simulink model "TestInSimulink"  (R2024b)
settings: Solver=FixedStepAuto  StartTime=0.0  StopTime=60.0  FixedStep=0.01  RelTol=1e-3
values from neighbouring files (symbols this model uses):
  DrivetrainEff = 0.95756    [TestInSimulink_prmts.m]
  Mode = 3    [TestInSimulink_prmts.m]
  Omega0 = 7.55    [TestInSimulink_prmts.m]
  rpm2radps = pi/30    (= 0.10471975512)    [TestInSimulink_prmts.m]
  SwingEq = 1/1836784*30/pi*1000    (= 0.00519892191216)    [TestInSimulink_prmts.m]
libraries: simulink x1
settings Model: Creator=valentinc  LastModifiedBy=valentinc
settings DebuggingCC: DebugExecutionForFMUViaOutOfProcess=on
settings RTWCC: GPUComputeCapability=3.5

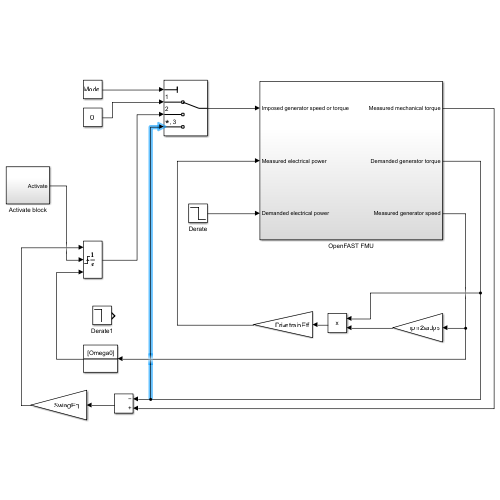
[thumbnail: Simulink's stored preview of the top-level diagram]
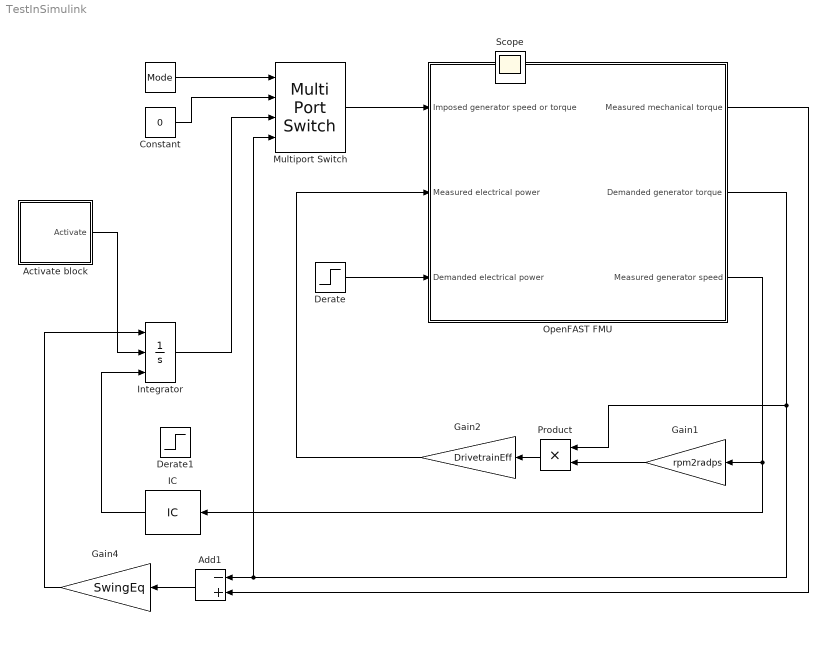
== system TestInSimulink ==
  " " : Constant  Value=Mode
  Activate block : Subsystem
  Add1 : Sum  Inputs=-+
  Constant : Constant  Value=0
  Derate : Step  Time=5  Before=2e4  After=1e4  SampleTime=0
  Derate1 : Step  Time=5  Before=19000  After=12000  SampleTime=0
  Gain1 : Gain  Gain=rpm2radps
  Gain2 : Gain  Gain=DrivetrainEff
  Gain4 : Gain  Gain=SwingEq
  IC : InitialCondition  Value=Omega0
  Integrator : Integrator  ExternalReset=rising  InitialConditionSource=external  InitialCondition=7.55
  Multiport Switch : MultiPortSwitch  SaturateOnIntegerOverflow=off  InputSameDT=off
  OpenFAST FMU : Subsystem
  Product : Product
  Scope : Scope
  wires:
  Product/1 -> Gain2/1
  Derate/1 -> OpenFAST FMU/3(Demanded electrical power)
  IC/1 -> Integrator/3
  Gain2/1 -> OpenFAST FMU/2(Measured electrical power)
  Gain1/1 -> Product/2
  OpenFAST FMU/3(Measured generator speed) -> Gain1/1, IC/1
  OpenFAST FMU/2(Demanded generator torque) -> Multiport Switch/4, Add1/1, Product/1
  Add1/1 -> Gain4/1
  Gain4/1 -> Integrator/1
  Activate block/1(Activate) -> Integrator/2
  " "/1 -> Multiport Switch/1
  Multiport Switch/1 -> OpenFAST FMU/1(Imposed generator speed or torque)
  Integrator/1 -> Multiport Switch/3
  OpenFAST FMU/1(Measured mechanical torque) -> Add1/2
  Constant/1 -> Multiport Switch/2

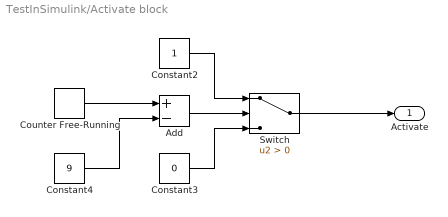
== system TestInSimulink/Activate block ==
  Add : Sum  Inputs=+-
  Constant2 : Constant
  Constant3 : Constant  Value=0
  Constant4 : Constant  Value=9
  Counter Free-Running : simulink/Sources/Counter Free-Running  NumBits=16  tsamp=-1
  Switch : Switch  Criteria=u2 > Threshold  SaturateOnIntegerOverflow=off  InputSameDT=off
  Activate : Outport
  wires:
  Constant2/1 -> Switch/1
  Constant4/1 -> Add/2
  Counter Free-Running/1 -> Add/1
  Add/1 -> Switch/2
  Constant3/1 -> Switch/3
  Switch/1 -> Activate/1

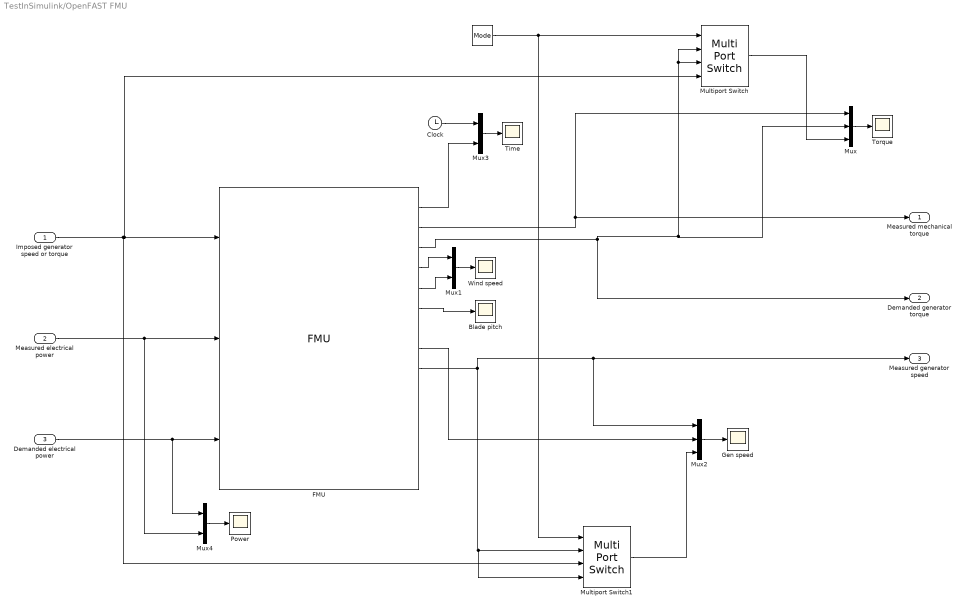
== system TestInSimulink/OpenFAST FMU ==
  Imposed generator speed or torque : Inport
  Measured electrical power : Inport  Port=2
  Demanded electrical power : Inport  Port=3
  "  " : Constant  Value=Mode
  Blade pitch : Scope
  Clock : Clock
  FMU : FMU  FMUName=fast.fmu  FMUDebugLogging=on  FMUMode=CoSimulation  FMUIsToleranceUsed=on  FMUSampleTime=0.01  FMUInitializeEnumObject=off  FMUCachedDialogLayout="{\"Geometry\":[2070,342,1033,905],\"ParameterColumnsWidthConfig\":\"{\\\"columns\\\":[{\\\"name\\\":\\\"Parameter\\\",\\\"width\\\":95},{\\\"name\\\":\\\"Value\\\",\\\"width\\\":59},{\\\"name\\\":\\\"Unit\\\",\\\"width\\\":49},{\\\"name\\\":\\\"Description\\\",\\\"width\\\":103}]}\",\"InputColumnsWidthConfig\":\"{\\\"columns\\\":[{\\\"name\\\":\\\"Name\\\",\\\"width\\\":63},{\\\"name\\\":\\\"Visibility\\\",\\\"width\\\":79},{\\\"name\\\":\\\"Start\\\",\\\"width\\\":52},{\\\"name\\\":\\\"Unit\\\",\\\"width\\\":49},{\\\"name\\\":\\\"Type Object\\\",\\\"width\\\":107}]}\",\"OutputColumnsWidthConfig\":\"{\\\"columns\\\":[{\\\"name\\\":\\\"Name\\\",\\\"width\\\":292},{\\\"name\\\":\\\"Visibility\\\",\\\"width\\\":79},{\\\"name\\\":\\\"Start\\\",\\\"width\\\":281},{\\\"name\\\":\\\"Unit\\\",\\\"width\\\":278},{\\\"name\\\":\\\"Type Object\\\",\\\"width\\\":337}]}\"}"  testNr=1002  timeStart=0  Mode=Mode  DebugPrmt=1  mask(FAST FMU [Co-Simulation, v2.0]){}
      mask Display:
      | disp('FAST FMU');
      | port_label('output',1,'Time');
      | port_label('output',2,'HSShftTq');
      | port_label('output',3,'GenTq');
      | port_label('output',4,'Wind1VelX');
      | port_label('output',5,'RtVAvgxh');
      | port_label('output',6,'BldPitch1');
      | port_label('output',7,'NacYaw');
      | port_label('output',8,'RefGenSpd');
      | port_label('output',9,'GenSpeed');
      | port_label('output',10,'RotSpeed');
      | port_label('output',11,'LSSGagPxa');
      | port_label('output',12,'Azimuth');
      | port_label('output',13,'GenAccel');
      | port_label('output',14,'YawBrTAxp');
      | port_label('input',1,'GenSpdOrTrq');
      | port_label('input',2,'GenPwr');
      | port_label('input',3,'ElecPwrCom');
  Gen speed : Scope
  Multiport Switch : MultiPortSwitch  SaturateOnIntegerOverflow=off  InputSameDT=off
  Multiport Switch1 : MultiPortSwitch  SaturateOnIntegerOverflow=off  InputSameDT=off
  Mux : Mux  Inputs=3
  Mux1 : Mux  Inputs=2
  Mux2 : Mux  Inputs=3
  Mux3 : Mux  Inputs=2
  Mux4 : Mux  Inputs=2
  Power : Scope
  Time : Scope
  Torque : Scope
  Wind speed : Scope
  Measured mechanical torque : Outport
  Demanded generator torque : Outport  Port=2
  Measured generator speed : Outport  Port=3
  wires:
  FMU/9 -> Mux2/1, Measured generator speed/1, Multiport Switch1/4, Multiport Switch1/2
  Demanded electrical power/1 -> Mux4/1, FMU/3
  Measured electrical power/1 -> Mux4/2, FMU/2
  FMU/3 -> Mux/2, Multiport Switch/3, Multiport Switch/2, Demanded generator torque/1
  FMU/2 -> Mux/1, Measured mechanical torque/1
  Mux/1 -> Torque/1
  FMU/6 -> Blade pitch/1
  FMU/4 -> Mux1/1
  FMU/5 -> Mux1/2
  Mux1/1 -> Wind speed/1
  FMU/8 -> Mux2/2
  Multiport Switch1/1 -> Mux2/3
  Mux2/1 -> Gen speed/1
  Imposed generator speed or torque/1 -> Multiport Switch1/3, Multiport Switch/4, FMU/1
  Mux4/1 -> Power/1
  Clock/1 -> Mux3/1
  FMU/1 -> Mux3/2
  Mux3/1 -> Time/1
  "  "/1 -> Multiport Switch1/1, Multiport Switch/1
  Multiport Switch/1 -> Mux/3
